simulink model "Invert_Pendulum"  (R2021b)
settings: Solver=VariableStepAuto  StartTime=0.0  StopTime=10  RelTol=1e-3
libraries: simulink x2, slpidlib x2
settings Model: Creator=15294  LastModifiedBy=15294

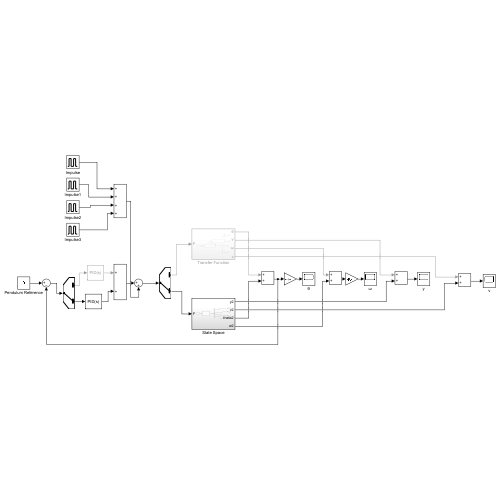
[thumbnail: Simulink's stored preview of the top-level diagram]
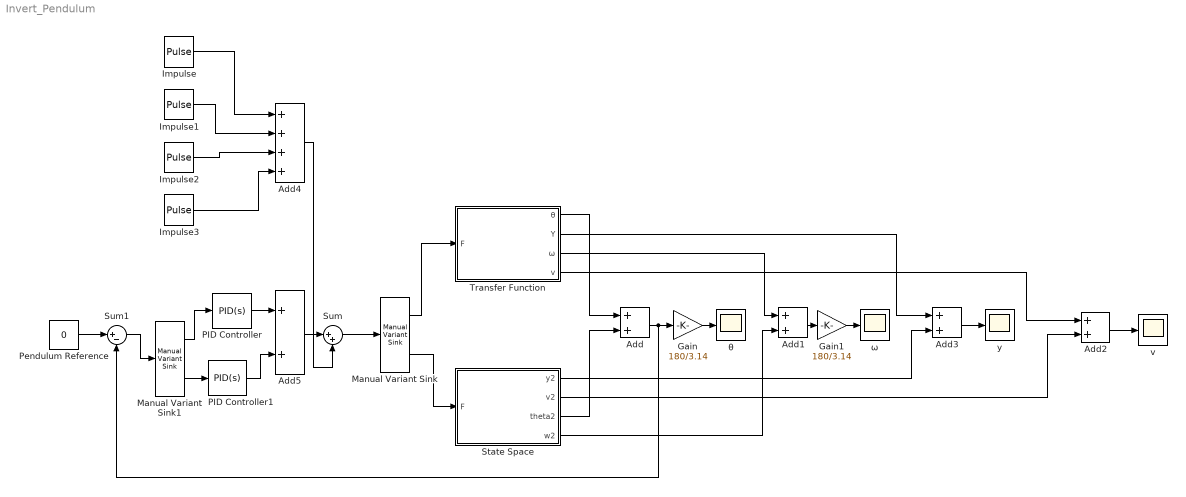
== system Invert_Pendulum ==
  Add{,1..3,5} (5 alike) : Sum
  Add4 : Sum  Inputs=++++
  Gain : Gain  Gain=180/3.14
  Gain1 : Gain  Gain=180/3.14
  Impulse : DiscretePulseGenerator  PulseType=Time based  Amplitude=10e5  Period=10  PulseWidth=0.01  PhaseDelay=2
  Impulse1 : DiscretePulseGenerator  PulseType=Time based  Amplitude=-10e5  Period=10  PulseWidth=0.01  PhaseDelay=4
  Impulse2 : DiscretePulseGenerator  PulseType=Time based  Amplitude=10e5  Period=10  PulseWidth=0.01  PhaseDelay=6
  Impulse3 : DiscretePulseGenerator  PulseType=Time based  Amplitude=-10e5  Period=10  PulseWidth=0.01  PhaseDelay=8
  Manual Variant Sink : simulink/Signal Routing/Manual Variant Sink  NumChoices=2  LabelModeActiveChoice=V_2
  Manual Variant Sink1 : simulink/Signal Routing/Manual Variant Sink  NumChoices=2  LabelModeActiveChoice=V_2
  PID Controller : slpidlib/PID Controller  Controller=PID  Form=Parallel  TimeDomain=Continuous-time  UseExternalTs=off  SampleTime=-1  IntegratorMethod=Forward Euler  FilterMethod=Forward Euler  ControllerParametersSource=internal  P=14606.6708911124  I=15948.6747414355  D=2916.27077260327  UseFilter=on  N=187.986393577918  TunerSelectOption=Transfer Function Based (PID Tuner App)  InitialConditionSource=internal  InitialConditionForIntegrator=0  InitialConditionForFilter=0  DifferentiatorICPrevScaledInput=0  ExternalReset=none  TrackingMode=off  Kt=1  LimitOutput=off  SatLimitsSource=internal  UpperSaturationLimit=inf  LowerSaturationLimit=-inf  LinearizeAsGain=on  AntiWindupMode=none  Kb=1  POutMin=[]  POutMax=[]  IOutMin=[]  IOutMax=[]  DOutMin=[]  DOutMax=[]  NOutMin=[]  NOutMax=[]  SumOutMin=[]  SumOutMax=[]  SaturationOutMin=[]  SaturationOutMax=[]  PParamMin=[]  PParamMax=[]  IParamMin=[]  IParamMax=[]  DParamMin=[]  DParamMax=[]  NParamMin=[]  NParamMax=[]  KbParamMin=[]  KbParamMax=[]  KtParamMin=[]  KtParamMax=[]  KbOutMin=[]  KbOutMax=[]  KtOutMin=[]  KtOutMax=[]  IntegratorOutMin=[]  IntegratorOutMax=[]  FilterOutMin=[]  FilterOutMax=[]  SumI1OutMin=[]  SumI1OutMax=[]  SumI2OutMin=[]  SumI2OutMax=[]  SumI3OutMin=[]  SumI3OutMax=[]  SumI4OutMin=[]  SumI4OutMax=[]  SumDOutMin=[]  SumDOutMax=[]  DifferentiatorOutMin=[]  DifferentiatorOutMax=[]  FilterDiffOutCoefMin=[]  FilterDiffOutCoefMax=[]  ReciprocalOutMin=[]  ReciprocalOutMax=[]  SumDenOutMin=[]  SumDenOutMax=[]  SumNumOutMin=[]  SumNumOutMax=[]  DivideOutMin=[]  DivideOutMax=[]  UdiffTsProdOutMin=[]  UdiffTsProdOutMax=[]  NTsProdOutMin=[]  NTsProdOutMax=[]  UintegralTsProdOutMin=[]  UintegralTsProdOutMax=[]  UngainTsProdOutMin=[]  UngainTsProdOutMax=[]  IntegratorContinuousStateAttributes=''  IntegratorStateMustResolveToSignalObject=off  IntegratorRTWStateStorageClass=Auto  FilterContinuousStateAttributes=''  FilterStateMustResolveToSignalObject=off  FilterRTWStateStorageClass=Auto  ParallelPVariant=InternalParameters  IdealPVariant=Disabled  IVariant=InternalParameters  DVariant=InternalParameters  IntegratorVariant=Continuous  SatVariant=Disabled  AWVariant=Passthrough  PCopyVariant=Disabled  TRVariant=Disabled  FdbkBlocksVariant=Forward  IdealPFdbkVariant=Disabled  SatFdbkVariant=Disabled  DerivativeFilterVariant=ContFilter  NVariant=InternalParameters  NCopyVariant=Disabled  FilterICVariant=InternalICsFilter  IntegratorICVariant=InternalICs  ExternalResetVariant=Disabled  TRSumVariant=Passthrough  SumFdbkVariant=Disabled  SumVariant=Sum_PID  TsampFilterVariant=InternalTs  TsampNgainVariant=Passthrough  TsampIntegralVariant=Passthrough  ExternalSaturationOutDataTypeStr=Inherit: Same as second input
  PID Controller1 : slpidlib/PID Controller  Controller=PID  Form=Parallel  TimeDomain=Continuous-time  UseExternalTs=off  SampleTime=-1  IntegratorMethod=Forward Euler  FilterMethod=Forward Euler  ControllerParametersSource=internal  P=-22479.718502026  I=-43244.7008553664  D=-2869.40683583955  UseFilter=on  N=224.115463401982  TunerSelectOption=Transfer Function Based (PID Tuner App)  InitialConditionSource=internal  InitialConditionForIntegrator=0  InitialConditionForFilter=0  DifferentiatorICPrevScaledInput=0  ExternalReset=none  TrackingMode=off  Kt=1  LimitOutput=off  SatLimitsSource=internal  UpperSaturationLimit=inf  LowerSaturationLimit=-inf  LinearizeAsGain=on  AntiWindupMode=none  Kb=1  POutMin=[]  POutMax=[]  IOutMin=[]  IOutMax=[]  DOutMin=[]  DOutMax=[]  NOutMin=[]  NOutMax=[]  SumOutMin=[]  SumOutMax=[]  SaturationOutMin=[]  SaturationOutMax=[]  PParamMin=[]  PParamMax=[]  IParamMin=[]  IParamMax=[]  DParamMin=[]  DParamMax=[]  NParamMin=[]  NParamMax=[]  KbParamMin=[]  KbParamMax=[]  KtParamMin=[]  KtParamMax=[]  KbOutMin=[]  KbOutMax=[]  KtOutMin=[]  KtOutMax=[]  IntegratorOutMin=[]  IntegratorOutMax=[]  FilterOutMin=[]  FilterOutMax=[]  SumI1OutMin=[]  SumI1OutMax=[]  SumI2OutMin=[]  SumI2OutMax=[]  SumI3OutMin=[]  SumI3OutMax=[]  SumI4OutMin=[]  SumI4OutMax=[]  SumDOutMin=[]  SumDOutMax=[]  DifferentiatorOutMin=[]  DifferentiatorOutMax=[]  FilterDiffOutCoefMin=[]  FilterDiffOutCoefMax=[]  ReciprocalOutMin=[]  ReciprocalOutMax=[]  SumDenOutMin=[]  SumDenOutMax=[]  SumNumOutMin=[]  SumNumOutMax=[]  DivideOutMin=[]  DivideOutMax=[]  UdiffTsProdOutMin=[]  UdiffTsProdOutMax=[]  NTsProdOutMin=[]  NTsProdOutMax=[]  UintegralTsProdOutMin=[]  UintegralTsProdOutMax=[]  UngainTsProdOutMin=[]  UngainTsProdOutMax=[]  IntegratorContinuousStateAttributes=''  IntegratorStateMustResolveToSignalObject=off  IntegratorRTWStateStorageClass=Auto  FilterContinuousStateAttributes=''  FilterStateMustResolveToSignalObject=off  FilterRTWStateStorageClass=Auto  ParallelPVariant=InternalParameters  IdealPVariant=Disabled  IVariant=InternalParameters  DVariant=InternalParameters  IntegratorVariant=Continuous  SatVariant=Disabled  AWVariant=Passthrough  PCopyVariant=Disabled  TRVariant=Disabled  FdbkBlocksVariant=Forward  IdealPFdbkVariant=Disabled  SatFdbkVariant=Disabled  DerivativeFilterVariant=ContFilter  NVariant=InternalParameters  NCopyVariant=Disabled  FilterICVariant=InternalICsFilter  IntegratorICVariant=InternalICs  ExternalResetVariant=Disabled  TRSumVariant=Passthrough  SumFdbkVariant=Disabled  SumVariant=Sum_PID  TsampFilterVariant=InternalTs  TsampNgainVariant=Passthrough  TsampIntegralVariant=Passthrough  ExternalSaturationOutDataTypeStr=Inherit: Same as second input
  Pendulum Reference : Constant  Value=0  OutDataTypeStr=Inherit: Inherit via back propagation
  State Space : Subsystem
  Sum : Sum  Inputs=|++
  Sum1 : Sum  Inputs=|+-
  Transfer Function : Subsystem
  v : Scope
  y : Scope
  θ : Scope
  ω : Scope
  wires:
  Pendulum Reference/1 -> Sum1/1
  Impulse/1 -> Add4/1
  Sum/1 -> Manual Variant Sink/1
  Manual Variant Sink/1 -> Transfer Function/1(F)
  Manual Variant Sink/2 -> State Space/1(F)
  Add/1 -> Sum1/2, Gain/1
  Add1/1 -> Gain1/1
  Add3/1 -> y/1
  Add2/1 -> v/1
  Impulse1/1 -> Add4/2
  Impulse2/1 -> Add4/3
  Impulse3/1 -> Add4/4
  Add4/1 -> Sum/2
  Transfer Function/1(θ) -> Add/1
  Transfer Function/2(Y) -> Add3/1
  Transfer Function/3(ω) -> Add1/1
  Transfer Function/4(v) -> Add2/1
  Gain/1 -> θ/1
  Gain1/1 -> ω/1
  Sum1/1 -> Manual Variant Sink1/1
  Manual Variant Sink1/1 -> PID Controller/1
  Manual Variant Sink1/2 -> PID Controller1/1
  PID Controller1/1 -> Add5/2
  PID Controller/1 -> Add5/1
  Add5/1 -> Sum/1
  State Space/1(y2) -> Add3/2
  State Space/2(v2) -> Add2/2
  State Space/3(theta2) -> Add/2
  State Space/4(w2) -> Add1/2

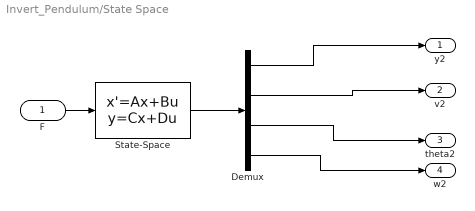
== system Invert_Pendulum/State Space ==
  F : Inport
  Demux : Demux
  State-Space : StateSpace  A=[0 1 0 0;0 0 -7.0335 0;0 0 0 1;0 0 14.853 0]  B=[0;0.016;0;-0.01407]  C=[1 0 0 0;0 1 0 0;0 0 1 0;0 0 0 1]  D=[0;0;0;0]  InitialCondition=0
  y2 : Outport
  v2 : Outport  Port=2
  theta2 : Outport  Port=3
  w2 : Outport  Port=4
  wires:
  F/1 -> State-Space/1
  Demux/4 -> w2/1
  Demux/1 -> y2/1
  Demux/3 -> theta2/1
  State-Space/1 -> Demux/1
  Demux/2 -> v2/1

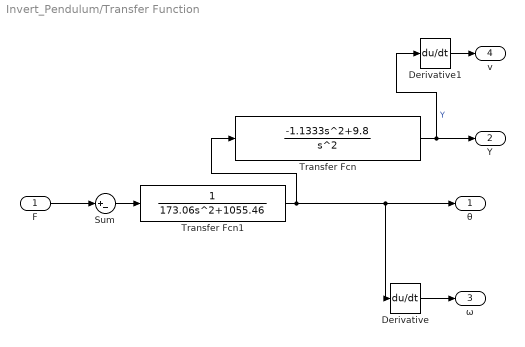
== system Invert_Pendulum/Transfer Function ==
  F : Inport
  Derivative : Derivative
  Derivative1 : Derivative
  Sum : Sum  Inputs=|+-
  Transfer Fcn : TransferFcn  Numerator=[-1.1333 0 9.8]  Denominator=[1 0 0]
  Transfer Fcn1 : TransferFcn  Denominator=[173.06 0 1055.46]
  θ : Outport
  Y : Outport  Port=2
  ω : Outport  Port=3
  v : Outport  Port=4
  wires:
  Sum/1 -> Transfer Fcn1/1
  Transfer Fcn/1 -> Derivative1/1, Y/1  "Y"
  F/1 -> Sum/1
  Transfer Fcn1/1 -> θ/1, Derivative/1, Transfer Fcn/1
  Derivative1/1 -> v/1
  Derivative/1 -> ω/1
